simulink library "WECSim_Lib_Moorings"  (R2020b)
settings: Solver=VariableStepAuto  StartTime=0.0  StopTime=10.0  RelTol=1e-3
undefined symbols (not defined in the file or in its folder): mooring, simu, X, Y, Z
libraries: sm_lib x10, nesl_utility x4, WECSim_Lib_Body_Elements x2
settings Model: Creator=kmruehl  LastModifiedBy=jtgrasb
settings DebuggingCC: SFMachineParentedDataDiag=error

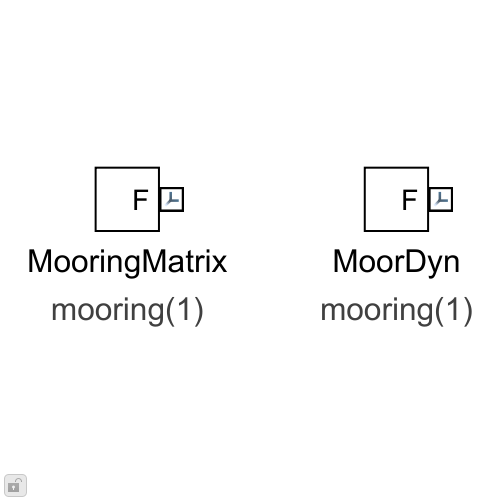
[thumbnail: Simulink's stored preview of the top-level diagram]
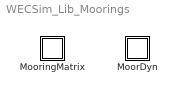
== system WECSim_Lib_Moorings ==
  MoorDyn : Subsystem  mask(MoorDyn){mooring=mooring(1), InputFileText=Global Reference Frame option "Use Input File" is selected., MooringRef=0  0  0, moorDynNodes=0, moorDynLines=0}
      mask prompts: mooring "Mooring Name:"; MooringRef "Reference Location [m]:"; moorDynNodes "Number of MoorDyn Nodes:"; moorDynLines "Number of MoorDyn Lines:"
      mask help:
      | A mooring body that applies stiffness, damping and pretensions forces to the follower using a MoorDyn simulation. The response of the mooring body is relative to the global reference frame.
      |
      | The variable name input below must be 'mooring(i)' where i=1,2,...
      | mooring(i) must be defined in the input file with the following fields:
      |
      |     .name (required)
      |             String.
      |             Mooring name. Must comply with Matlab's variable naming rules.
      |     .location (optional)
      |             3x1 vector [x y z] in meters.
      |             Mooring location. Default = [0 0 0]
      |     .initial (optional)
      |             Struct
      |             Contains the initial position, angle and axis of the mooring body.
      |     .initial.displacement (optional)
      |             3x1 vector [x y z] in meters.
      |             Initial linear displacement from the ref position. Default = [0 0 0]
      |             This can can be set directly or with the setInitDisp() method.
      |     .initial.axis (optional)
      |             3x1 vector [x y z]
      |             Initial angular displacement axis. Default = [0 1 0]
      |             This can can be set directly or with the setInitDisp() method.
      |     .initial.angle (optional)
      |             Float.
      |             Initial angular displacement angle about axis in radians. Default = [0 0 0]
      |             This can can be set directly or with the setInitDisp() method.
      |     .moorDynLines (optional)
      |             Float.
      |             Number of lines for MoorDyn to use. Default = 0
      |     .moorDynNodes (optional)
      |             moorDynLines x 1 vector.
      |             Specifies the number of nodes per line in MoorDyn. Default = []
      mask init:
      | if exist('mooring','var')
      |     % toWorkSpace: outputs
      |     h=[gcb '/To Workspace'];
      |     responseName=['mooring' num2str(mooring.number) '_out'];
      |     set_param(h,'VariableName',responseName);
      | end
      | mooring.moorDyn = 1;
      settings: AttributesFormatString=%<mooring>
      mask Help:
      | A mooring body that applies stiffness, damping and pretensions forces to the follower using a MoorDyn simulation. The response of the mooring body is relative to the global reference frame.
      | 
      | The variable name input below must be 'mooring(i)' where i=1,2,...
      | mooring(i) must be defined in the input file with the following fields:
      | 
      |     .name (required)
      |             String.
      |             Mooring name. Must comply with Matlab's variable naming rules.
      |     .location (optional)
      |             3x1 vector [x y z] in meters.
      |             Mooring location. Default = [0 0 0]
      |     .initial (optional)
      |             Struct
      |             Contains the initial position, angle and axis of the mooring body.
      |     .initial.displacement (optional)
      |             3x1 vector [x y z] in meters.
      |             Initial linear displacement from the ref position. Default = [0 0 0]
      |             This can can be set directly or with the setInitDisp() method.
      |     .initial.axis (optional)
      |             3x1 vector [x y z]
      |             Initial angular displacement axis. Default = [0 1 0]
      |             This can can be set directly or with the setInitDisp() method.
      |     .initial.angle (optional)
      |             Float.
      |             Initial angular displacement angle about axis in radians. Default = [0 0 0]
      |             This can can be set directly or with the setInitDisp() method.
      |     .moorDynLines (optional)
      |             Float.
      |             Number of lines for MoorDyn to use. Default = 0
      |     .moorDynNodes (optional)
      |             moorDynLines x 1 vector.
      |             Specifies the number of nodes per line in MoorDyn. Default = []
      mask DialogControl InputFileGroup Prompt: Input File
      mask DialogControl CustomParameterGroup Prompt: Custom Parameters
  MooringMatrix : Subsystem  mask(Mooring Matrix){mooring=mooring(1), InputFileText=Global Reference Frame option "Use Input File" is selected., loc=0 0 0, preTension=[0 0 0 0 0 0], stiffness={ '0', '0', '0', '0', '0', '0'; '0', '0', '0', '0', '0', '0'; '0', '0', '0', '0', '0', '0'; '0', '0', '0', '0', '0', '0'; '0', '0', '0', '0', '0', '0'; '0', '0', '0', '0', '0', '0' }, damping={ '0', '0', '0', '0', '0', '0'; '0', '0', '0', '0', '0', '0'; '0', '0', '0', '0', '0', '0'; '0', '0', '0', '0', '0', '0'; '0', '0', '0', '0', '0', '0'; '0', '0', '0', '0', '0', '0' }}
      mask prompts: mooring "Mooring Name:"; loc "Reference Location [m]:"; preTension "Pretension Force [N]:"; stiffness "Stiffness [N/m]:"; damping "Damping [N/m^2]:"
      mask help:
      | A mooring body that applies stiffness, damping and pretensions forces to the follower. The response of the mooring body is relative to the global reference frame.
      |
      | The variable name input below must be 'mooring(i)' where i=1,2,...
      | mooring(i) must be defined in the input file with the following fields:
      |
      |     .name (required)
      |             String.
      |             Mooring name. Must comply with Matlab's variable naming rules.
      |     .location (optional)
      |             3x1 vector [x y z] in meters.
      |             Mooring location. Default = [0 0 0]
      |     .initial (optional)
      |             Struct
      |             Contains the initial position, angle and axis of the mooring body.
      |     .initial.displacement (optional)
      |             3x1 vector [x y z] in meters.
      |             Initial linear displacement from the ref position. Default = [0 0 0]
      |             This can can be set directly or with the setInitDisp() method.
      |     .initial.axis (optional)
      |             3x1 vector [x y z]
      |             Initial angular displacement axis. Default = [0 1 0]
      |             This can can be set directly or with the setInitDisp() method.
      |     .initial.angle (optional)
      |             Float.
      |             Initial angular displacement angle about axis in radians. Default = [0 0 0]
      |             This can can be set directly or with the setInitDisp() method.
      |     .matrix (optional)
      |             Struct
      |             Contains the stiffness matrix, damping matrix and pretension of the mooring body.
      |     .matrix.stiffness (optional)
      |             6x6 vector.
      |             Mooring linear spring stiffness. Default = zeros(6)
      |     .matrix.damping (optional)
      |             6x6 vector.
      |             Mooring linear damping coefficient. Default = zeros(6)
      |     .matrix.preTension (optional)
      |             6x1 vector.
      |             Mooring preTension force. Default = [0 0 0 0 0 0]
      mask init:
      | if exist('mooring','var')
      |     % toWorkSpace: outputs
      |     h=[gcb '/To Workspace'];
      |     responseName=['mooring' num2str(mooring.number) '_out'];
      |     set_param(h,'VariableName',responseName);
      | end
      settings: AttributesFormatString=%<mooring>
      mask Help:
      | A mooring body that applies stiffness, damping and pretensions forces to the follower. The response of the mooring body is relative to the global reference frame.
      | 
      | The variable name input below must be 'mooring(i)' where i=1,2,...
      | mooring(i) must be defined in the input file with the following fields:
      | 
      |     .name (required)
      |             String.
      |             Mooring name. Must comply with Matlab's variable naming rules.
      |     .location (optional)
      |             3x1 vector [x y z] in meters.
      |             Mooring location. Default = [0 0 0]
      |     .initial (optional)
      |             Struct
      |             Contains the initial position, angle and axis of the mooring body.
      |     .initial.displacement (optional)
      |             3x1 vector [x y z] in meters.
      |             Initial linear displacement from the ref position. Default = [0 0 0]
      |             This can can be set directly or with the setInitDisp() method.
      |     .initial.axis (optional)
      |             3x1 vector [x y z]
      |             Initial angular displacement axis. Default = [0 1 0]
      |             This can can be set directly or with the setInitDisp() method.
      |     .initial.angle (optional)
      |             Float.
      |             Initial angular displacement angle about axis in radians. Default = [0 0 0]
      |             This can can be set directly or with the setInitDisp() method.
      |     .matrix (optional)
      |             Struct
      |             Contains the stiffness matrix, damping matrix and pretension of the mooring body.
      |     .matrix.stiffness (optional)
      |             6x6 vector.
      |             Mooring linear spring stiffness. Default = zeros(6)
      |     .matrix.damping (optional)
      |             6x6 vector.
      |             Mooring linear damping coefficient. Default = zeros(6)
      |     .matrix.preTension (optional)
      |             6x1 vector.
      |             Mooring preTension force. Default = [0 0 0 0 0 0]
      mask DialogControl InputFileGroup Prompt: Input File
      mask DialogControl CustomParameterGroup Prompt: Custom Parameters
      mask DialogControl matrix Prompt: Additional Parameters

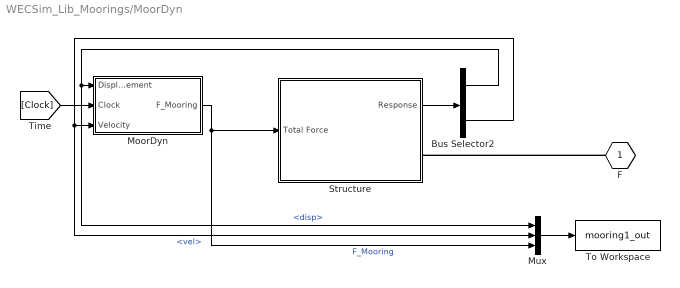
== system WECSim_Lib_Moorings/MoorDyn ==
  Bus Selector2 : BusSelector  OutputSignals=disp,vel
  MoorDyn : Subsystem  VariantControl=sv_moorDyn
  Mux : Mux  Inputs=3
  Structure : Subsystem
  To Workspace : ToWorkspace  VariableName=mooring1_out  SaveFormat=Structure With Time  SampleTime=simu.dtOut
  F : PMIOPort  Side=Left
  wires:
  Structure/1(Response) -> Bus Selector2/1
  MoorDyn/1(F_Mooring) -> Mux/3, Structure/1(Total Force)  "F_Mooring"
  [Clock] -> MoorDyn/2(Clock)
  Bus Selector2/1 -> Mux/1, MoorDyn/1(Displacement)  "<disp>"
  Bus Selector2/2 -> Mux/2, MoorDyn/3(Velocity)  "<vel>"
  Mux/1 -> To Workspace/1
  connections:
  F/RConn1 -- Structure/RConn1

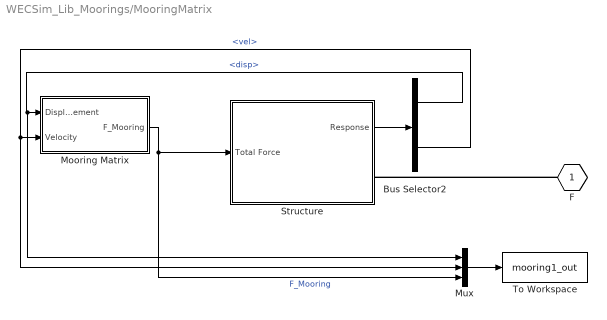
== system WECSim_Lib_Moorings/MooringMatrix ==
  Bus Selector2 : BusSelector  OutputSignals=disp,vel
  Mooring Matrix : Subsystem  VariantControl=sv_mooringMatrix
  Mux : Mux  Inputs=3
  Structure : Subsystem
  To Workspace : ToWorkspace  VariableName=mooring1_out  SaveFormat=Structure With Time  SampleTime=simu.dtOut
  F : PMIOPort  Side=Left
  wires:
  Structure/1(Response) -> Bus Selector2/1
  Mooring Matrix/1(F_Mooring) -> Mux/3, Structure/1(Total Force)  "F_Mooring"
  Bus Selector2/1 -> Mux/1, Mooring Matrix/1(Displacement)  "<disp>"
  Bus Selector2/2 -> Mux/2, Mooring Matrix/2(Velocity)  "<vel>"
  Mux/1 -> To Workspace/1
  connections:
  F/RConn1 -- Structure/RConn1

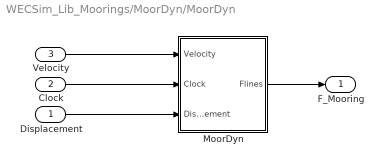
== system WECSim_Lib_Moorings/MoorDyn/MoorDyn ==
  Displacement : Inport
  Clock : Inport  Port=2
  Velocity : Inport  Port=3
  MoorDyn : Subsystem  InitFcn=|  StopFcn=|
      InitFcn=|
      | % Initialize MoorDyn Lib (Windows:dll or OSX:dylib)
      | disp('---------------Starting MoorDyn-----------')
      | 
      | if libisloaded('libmoordyn')
      |     calllib('libmoordyn', 'MoorDynClose');
      |     unloadlibrary libmoordyn;
      | end
      | 
      | if ismac
      |     loadlibrary('libmoordyn.dylib','MoorDyn.h');
      | elseif ispc
      |     loadlibrary('libmoordyn.dll','MoorDyn.h');
      | elseif isunix
      |     loadlibrary('libmoordyn.so','MoorDyn.h');
      | else
      |     disp('Cannot run MoorDyn in this platform');
      | end
      | 
      | calllib('libmoordyn', 'MoorDynInit', mooring.orientation, [0 0 0 0 0 0], mooring.moorDynInputFile);
      | disp('MoorDyn Initialized. Now time stepping...')
      StopFcn=|
      | calllib('libmoordyn', 'MoorDynClose');
      | unloadlibrary libmoordyn;
      settings: CloseFcn=|
      | calllib('libmoordyn', 'MoorDynClose');
      | unloadlibrary libmoordyn;
  F_Mooring : Outport
  wires:
  MoorDyn/1(Flines) -> F_Mooring/1
  Clock/1 -> MoorDyn/2(Clock)
  Displacement/1 -> MoorDyn/3(Displacement)
  Velocity/1 -> MoorDyn/1(Velocity)

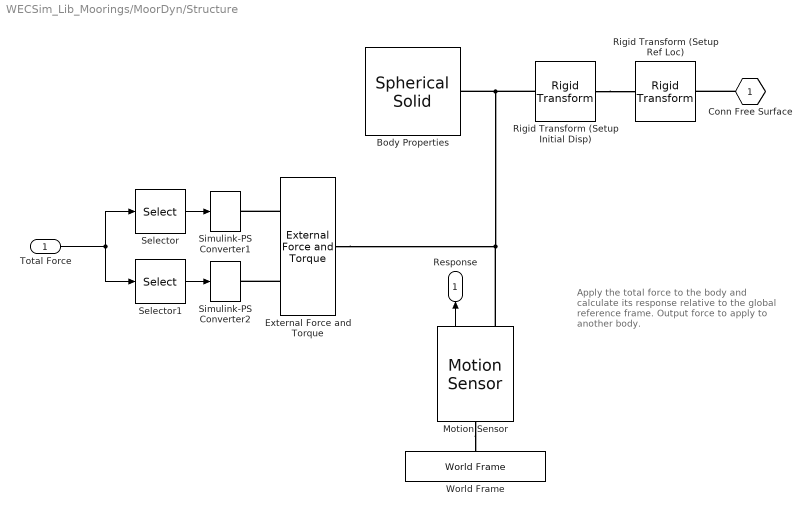
== system WECSim_Lib_Moorings/MoorDyn/Structure ==
  note: Apply the total force to the body and calculate its response relative to the global reference frame.
      |
      | Output force to apply to another body.
  Total Force : Inport
  Body Properties : sm_lib/Body Elements/Spherical Solid  GraphicAmbientColor=[0.15 0.15 0.15 1.0]  BasedOnType=Density  CenterOfMass=[0 0 0]  CenterOfMassUnits=m  GraphicDiffuseColor=[0 1 0]  Density=1000  DensityUnits=kg/(m^3)  DoExposeReferenceFrame=on  GraphicEmissiveColor=[0.0 0.0 0.0 1.0]  ExportEntireGeometry=off  SerializedExposedGeometries=<ExposedGeometries/>  SerializedFrames=<Frames/>  MarkerShape=Sphere  MarkerSize=10  GraphicType=None  InertiaType=Custom  Mass=0  MassUnits=kg  MomentsOfInertia=[0 0 0]  MomentsOfInertiaUnits=kg*m^2  GraphicOpacity=1  ProductsOfInertia=[0 0 0]  ProductsOfInertiaUnits=kg*m^2  GraphicShininess=75  GraphicSpecularColor=[0.5 0.5 0.5 1.0]  SphereRadius=1  SphereRadiusUnits=m  GraphicVisPropType=SimpleVisualProperties
  External Force and Torque : sm_lib/Forces and Torques/External Force and Torque  ForceResolutionFrame=World  EnableForceX=off  EnableForceY=off  EnableForceZ=off  EnableForce=on  TorqueResolutionFrame=World  EnableTorqueX=off  EnableTorqueY=off  EnableTorqueZ=off  EnableTorque=on
  Motion Sensor : WECSim_Lib_Body_Elements/Rigid Body/Hydrodynamic Body/Structure/Motion Sensor  SystemSampleTime=-1  VariantActivationTime=update diagram  Latency=0  AutoFrameSizeCalculation=off
  Rigid Transform (Setup Initial Disp) : sm_lib/Frames and Transforms/Rigid Transform  TranslationMethod=Cartesian  TranslationStandardOffset=0  TranslationLengthUnit=m  TranslationStandardAxis=+Z  TranslationCartesianOffset=mooring.initial.displacement  TranslationROffset=0  TranslationROffsetUnits=m  TranslationZOffset=0  TranslationZOffsetUnits=m  TranslationThetaOffset=0  TranslationThetaOffsetUnits=deg  RotationMethod=ArbitraryAxis  RotationAngleUnits=rad  RotationStandardAxis=+Y  RotationAngle=mooring.initial.angle  RotationArbitraryAxis=mooring.initial.axis  FollAlignAxisA=+X  BaseAlignAxisA=+Y  FollAlignAxisB=+Y  BaseAlignAxisB=+Z  RotationSequenceAxes=FollowerAxes  RotationSequence=XYX  RotationSequenceAngles=[0 0 0]  RotationSequenceAnglesUnits=deg  RotationMatrix=[1 0 0; 0 1 0; 0 0 1]  Quaternion=[1 0 0 0]
  Rigid Transform (Setup Ref Loc) : sm_lib/Frames and Transforms/Rigid Transform  TranslationMethod=Cartesian  TranslationStandardOffset=0  TranslationLengthUnit=m  TranslationStandardAxis=+Z  TranslationCartesianOffset=mooring.location  TranslationROffset=0  TranslationROffsetUnits=m  TranslationZOffset=0  TranslationZOffsetUnits=m  TranslationThetaOffset=0  TranslationThetaOffsetUnits=deg  RotationMethod=None  RotationAngleUnits=rad  RotationStandardAxis=+Y  RotationAngle=0.05  RotationArbitraryAxis=[0.57735026918962584 0.57735026918962584 0.57735026918962584]  FollAlignAxisA=+X  BaseAlignAxisA=+Y  FollAlignAxisB=+Y  BaseAlignAxisB=+Z  RotationSequenceAxes=FollowerAxes  RotationSequence=XYX  RotationSequenceAngles=[0 0 0]  RotationSequenceAnglesUnits=deg  RotationMatrix=[1 0 0; 0 1 0; 0 0 1]  Quaternion=[1 0 0 0]
  Selector : Selector  InputPortWidth=6  IndexOptions=Index vector (dialog)  Indices=[1:3]  OutputSizes=1
  Selector1 : Selector  InputPortWidth=6  IndexOptions=Index vector (dialog)  Indices=[4:6]  OutputSizes=1
  Simulink-PS Converter1 : nesl_utility/Simulink-PS Converter  PhysicalDomain=network_engine_domain  SubClassName=ps_input  LeftPortType=input  RightPortType=output  PseudoPeriodic=off  Frequencies=[]  NoiseDistribution=none  NoiseParameters=[]  Unit=1  AffineConversion=off  FilteringAndDerivatives=zero  SimscapeFilterOrder=1  InputFilterTimeConstant=0.001  UdotUserProvided=1
  Simulink-PS Converter2 : nesl_utility/Simulink-PS Converter  PhysicalDomain=network_engine_domain  SubClassName=ps_input  LeftPortType=input  RightPortType=output  PseudoPeriodic=off  Frequencies=[]  NoiseDistribution=none  NoiseParameters=[]  Unit=1  AffineConversion=off  FilteringAndDerivatives=zero  SimscapeFilterOrder=1  InputFilterTimeConstant=0.001  UdotUserProvided=1
  World Frame : sm_lib/Frames and Transforms/World Frame
  Conn Free Surface : PMIOPort  Side=Right
  Response : Outport
  wires:
  Total Force/1 -> Selector1/1, Selector/1
  Selector/1 -> Simulink-PS Converter1/1
  Selector1/1 -> Simulink-PS Converter2/1
  Motion Sensor/1 -> Response/1
  connections:
  External Force and Torque/LConn1 -- Simulink-PS Converter1/RConn1
  External Force and Torque/LConn2 -- Simulink-PS Converter2/RConn1
  Rigid Transform (Setup Initial Disp)/RConn1 -- Body Properties/RConn1 -- Motion Sensor/RConn1 -- External Force and Torque/RConn1
  Conn Free Surface/RConn1 -- Rigid Transform (Setup Ref Loc)/LConn1
  Rigid Transform (Setup Initial Disp)/LConn1 -- Rigid Transform (Setup Ref Loc)/RConn1
  Motion Sensor/LConn1 -- World Frame/RConn1

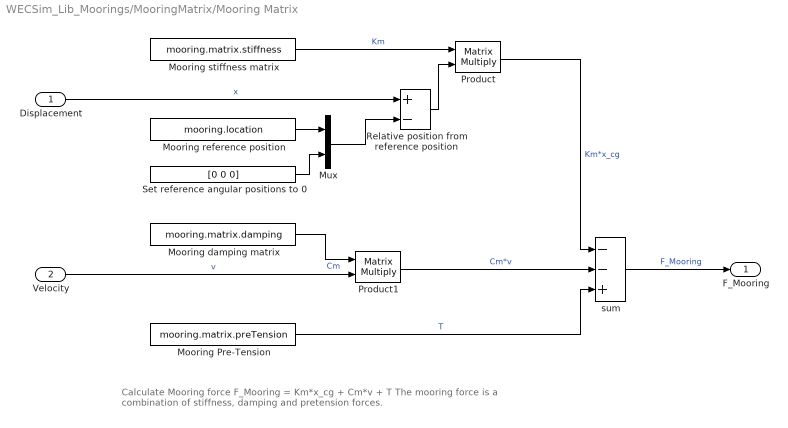
== system WECSim_Lib_Moorings/MooringMatrix/Mooring Matrix ==
  note: Calculate Mooring force
      |
      | F_Mooring = Km*x_cg + Cm*v + T
      | The mooring force is a combination of stiffness, damping and pretension forces.
  Displacement : Inport
  Velocity : Inport  Port=2
  Mooring Pre-Tension : Constant  Value=mooring.matrix.preTension
  Mooring damping matrix : Constant  Value=mooring.matrix.damping
  Mooring reference position : Constant  Value=mooring.location
  Mooring stiffness matrix : Constant  Value=mooring.matrix.stiffness
  Mux : Mux  Inputs=2
  Product : Product  Multiplication=Matrix(*)
  Product1 : Product  Multiplication=Matrix(*)
  Relative position from reference position : Sum  Inputs=+-
  Set reference angular positions to 0 : Constant  Value=[0 0 0]
  sum : Sum  Inputs=--+
  F_Mooring : Outport
  wires:
  Product/1 -> sum/1  "Km*x_cg"
  Product1/1 -> sum/2  "Cm*v"
  sum/1 -> F_Mooring/1  "F_Mooring"
  Mooring Pre-Tension/1 -> sum/3  "T"
  Mooring stiffness matrix/1 -> Product/1  "Km"
  Velocity/1 -> Product1/2  "v"
  Mooring damping matrix/1 -> Product1/1  "Cm"
  Displacement/1 -> Relative position from reference position/1  "x"
  Mooring reference position/1 -> Mux/1
  Set reference angular positions to 0/1 -> Mux/2
  Mux/1 -> Relative position from reference position/2
  Relative position from reference position/1 -> Product/2

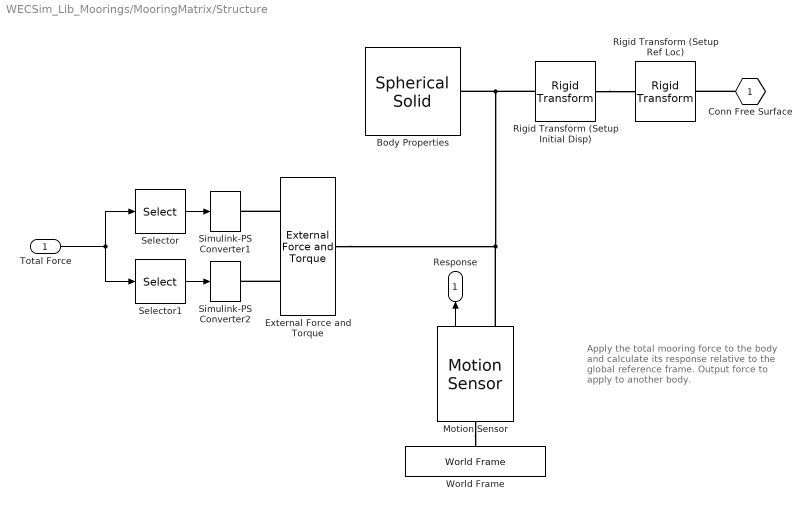
== system WECSim_Lib_Moorings/MooringMatrix/Structure ==
  note: Apply the total mooring force to the body and calculate its response relative to the global reference frame.
      |
      | Output force to apply to another body.
  Total Force : Inport
  Body Properties : sm_lib/Body Elements/Spherical Solid  GraphicAmbientColor=[0.15 0.15 0.15 1.0]  BasedOnType=Density  CenterOfMass=[0 0 0]  CenterOfMassUnits=m  GraphicDiffuseColor=[0 1 0]  Density=1000  DensityUnits=kg/(m^3)  DoExposeReferenceFrame=on  GraphicEmissiveColor=[0.0 0.0 0.0 1.0]  ExportEntireGeometry=off  SerializedExposedGeometries=<ExposedGeometries/>  SerializedFrames=<Frames/>  MarkerShape=Sphere  MarkerSize=10  GraphicType=None  InertiaType=Custom  Mass=0  MassUnits=kg  MomentsOfInertia=[0 0 0]  MomentsOfInertiaUnits=kg*m^2  GraphicOpacity=1  ProductsOfInertia=[0 0 0]  ProductsOfInertiaUnits=kg*m^2  GraphicShininess=75  GraphicSpecularColor=[0.5 0.5 0.5 1.0]  SphereRadius=1  SphereRadiusUnits=m  GraphicVisPropType=SimpleVisualProperties
  External Force and Torque : sm_lib/Forces and Torques/External Force and Torque  ForceResolutionFrame=World  EnableForceX=off  EnableForceY=off  EnableForceZ=off  EnableForce=on  TorqueResolutionFrame=World  EnableTorqueX=off  EnableTorqueY=off  EnableTorqueZ=off  EnableTorque=on
  Motion Sensor : WECSim_Lib_Body_Elements/Rigid Body/Hydrodynamic Body/Structure/Motion Sensor  SystemSampleTime=-1  VariantActivationTime=update diagram  Latency=0  AutoFrameSizeCalculation=off
  Rigid Transform (Setup Initial Disp) : sm_lib/Frames and Transforms/Rigid Transform  TranslationMethod=Cartesian  TranslationStandardOffset=0  TranslationLengthUnit=m  TranslationStandardAxis=+Z  TranslationCartesianOffset=mooring.initial.displacement  TranslationROffset=0  TranslationROffsetUnits=m  TranslationZOffset=0  TranslationZOffsetUnits=m  TranslationThetaOffset=0  TranslationThetaOffsetUnits=deg  RotationMethod=ArbitraryAxis  RotationAngleUnits=rad  RotationStandardAxis=+Y  RotationAngle=mooring.initial.angle  RotationArbitraryAxis=mooring.initial.axis  FollAlignAxisA=+X  BaseAlignAxisA=+Y  FollAlignAxisB=+Y  BaseAlignAxisB=+Z  RotationSequenceAxes=FollowerAxes  RotationSequence=XYX  RotationSequenceAngles=[0 0 0]  RotationSequenceAnglesUnits=deg  RotationMatrix=[1 0 0; 0 1 0; 0 0 1]  Quaternion=[1 0 0 0]
  Rigid Transform (Setup Ref Loc) : sm_lib/Frames and Transforms/Rigid Transform  TranslationMethod=Cartesian  TranslationStandardOffset=0  TranslationLengthUnit=m  TranslationStandardAxis=+Z  TranslationCartesianOffset=mooring.location  TranslationROffset=0  TranslationROffsetUnits=m  TranslationZOffset=0  TranslationZOffsetUnits=m  TranslationThetaOffset=0  TranslationThetaOffsetUnits=deg  RotationMethod=None  RotationAngleUnits=rad  RotationStandardAxis=+Y  RotationAngle=0.05  RotationArbitraryAxis=[0.57735026918962584 0.57735026918962584 0.57735026918962584]  FollAlignAxisA=+X  BaseAlignAxisA=+Y  FollAlignAxisB=+Y  BaseAlignAxisB=+Z  RotationSequenceAxes=FollowerAxes  RotationSequence=XYX  RotationSequenceAngles=[0 0 0]  RotationSequenceAnglesUnits=deg  RotationMatrix=[1 0 0; 0 1 0; 0 0 1]  Quaternion=[1 0 0 0]
  Selector : Selector  InputPortWidth=6  IndexOptions=Index vector (dialog)  Indices=[1:3]  OutputSizes=1
  Selector1 : Selector  InputPortWidth=6  IndexOptions=Index vector (dialog)  Indices=[4:6]  OutputSizes=1
  Simulink-PS Converter1 : nesl_utility/Simulink-PS Converter  PhysicalDomain=network_engine_domain  SubClassName=ps_input  LeftPortType=input  RightPortType=output  PseudoPeriodic=off  Frequencies=[]  NoiseDistribution=none  NoiseParameters=[]  Unit=1  AffineConversion=off  FilteringAndDerivatives=zero  SimscapeFilterOrder=1  InputFilterTimeConstant=0.001  UdotUserProvided=1
  Simulink-PS Converter2 : nesl_utility/Simulink-PS Converter  PhysicalDomain=network_engine_domain  SubClassName=ps_input  LeftPortType=input  RightPortType=output  PseudoPeriodic=off  Frequencies=[]  NoiseDistribution=none  NoiseParameters=[]  Unit=1  AffineConversion=off  FilteringAndDerivatives=zero  SimscapeFilterOrder=1  InputFilterTimeConstant=0.001  UdotUserProvided=1
  World Frame : sm_lib/Frames and Transforms/World Frame
  Conn Free Surface : PMIOPort  Side=Right
  Response : Outport
  wires:
  Total Force/1 -> Selector1/1, Selector/1
  Selector/1 -> Simulink-PS Converter1/1
  Selector1/1 -> Simulink-PS Converter2/1
  Motion Sensor/1 -> Response/1
  connections:
  External Force and Torque/LConn1 -- Simulink-PS Converter1/RConn1
  External Force and Torque/LConn2 -- Simulink-PS Converter2/RConn1
  Rigid Transform (Setup Initial Disp)/RConn1 -- Body Properties/RConn1 -- Motion Sensor/RConn1 -- External Force and Torque/RConn1
  Conn Free Surface/RConn1 -- Rigid Transform (Setup Ref Loc)/LConn1
  Rigid Transform (Setup Initial Disp)/LConn1 -- Rigid Transform (Setup Ref Loc)/RConn1
  Motion Sensor/LConn1 -- World Frame/RConn1

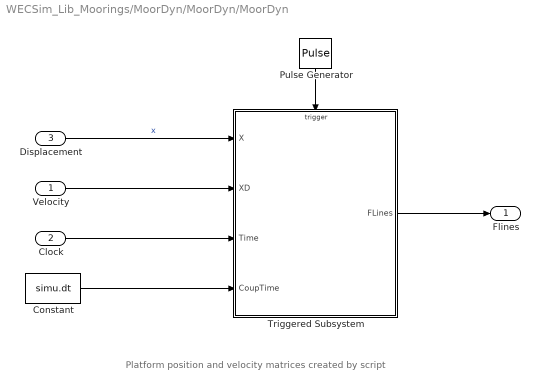
== system WECSim_Lib_Moorings/MoorDyn/MoorDyn/MoorDyn ==
  note: Platform position and velocity matrices created by script
  Velocity : Inport
  Clock : Inport  Port=2
  Displacement : Inport  Port=3
  Constant : Constant  Value=simu.dt
  Pulse Generator : DiscretePulseGenerator  PulseType=Time based  Amplitude=simu.endTime  Period=2*simu.dt  PulseWidth=50
  Triggered Subsystem : Subsystem  TreatAsAtomicUnit=on
  Flines : Outport
  wires:
  Displacement/1 -> Triggered Subsystem/1(X)  "x"
  Triggered Subsystem/1(FLines) -> Flines/1
  Clock/1 -> Triggered Subsystem/3(Time)
  Velocity/1 -> Triggered Subsystem/2(XD)
  Constant/1 -> Triggered Subsystem/4(CoupTime)
  Pulse Generator/1 -> Triggered Subsystem/Trigger

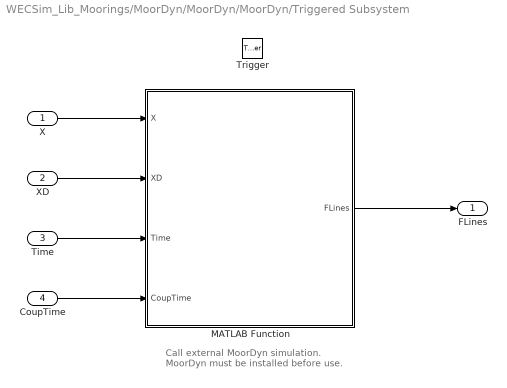
== system WECSim_Lib_Moorings/MoorDyn/MoorDyn/MoorDyn/Triggered Subsystem ==
  note: Call external MoorDyn simulation. MoorDyn must be installed before use.
  X : Inport
  XD : Inport  Port=2
  Time : Inport  Port=3
  CoupTime : Inport  Port=4
  Trigger : TriggerPort  TriggerType=either  VariantControl=(inherit)
  MATLAB Function : MATLAB Function  TreatAsAtomicUnit=on
  FLines : Outport  PortDimensions=6
  wires:
  CoupTime/1 -> MATLAB Function/4(CoupTime)
  Time/1 -> MATLAB Function/3(Time)
  XD/1 -> MATLAB Function/2(XD)
  MATLAB Function/1(FLines) -> FLines/1
  X/1 -> MATLAB Function/1(X)

== matlab function WECSim_Lib_Moorings/MoorDyn/MoorDyn/MoorDyn/Triggered Subsystem/MATLAB Function ==
  data: X input; FLines output; XD input; Time input; CoupTime input
function FLines  = MoorDyn_matlab_FCN(X,XD,Time,CoupTime)

FLines = zeros(1,6);
FLines  = MoorDyn_matlab_FCN(X,XD,Time,CoupTime);

end
